simulink model "Design_of_an_Energy_Efficient_Hybrid_Electric_Vehicle"  (R2023a)
settings: Solver=FixedStepDiscrete  StartTime=0  StopTime=110  RelTol=1e-3  EnableMultiTasking=on
PreLoadFcn:
  | power_motordrive_IPMSM_FOC_data
InitFcn:
  | power_motordrive_IPMSM_FOC_data
  | Cdc  = 0.001;      % DC-link capacitor  [F]
  | AH0  = 280;        % Initial battery charge [hr*A]
  | Tmax=410;
  | 
  | %% Vehicle Parameters for Vehicle Dynamics 2
  | vehicle_mass = 2111;
  | wheel_radius = 0.228;
  | area =2.22;
  | drag_coefficient = 0.23;
  | air_density = 1.204;
  | gravity = 9.81;
  | rolling_res_ratio = 0.02;
  | 
  | % Differential drive parameters
  | gear_ratio = 5;
  | i_t   = gear_ratio ;
  | Rw=wheel_radius;
  | 
  | 
  | %% Sliding Mode Observer
  | pmsm.N_max=wmax;
  | pmsm.p=p
  | pmsm.Ld=Ld;
  | pmsm.Lq=Lq;
  | pmsm.Rs=Rs;
  | PU_System.V_base=(Vdc_nom/sqrt(3));
  | PU_System.I_base=lambda/(Lq-Ld);
  | max_torque=400
  | force_max_pedal=500
  | braking_torque_to_pedal_force_ratio=-4
undefined symbols (not defined in the file): BlkSampleTime, CurrentObserverGain, dataType, DiscIntNeverNeededParam, Fsw, gcbh, Ki_Ireg, Ki_wreg, Kp_Ireg, Kp_wreg, L_smo_gain, lambda, Ld, Limit_Ireg, Limit_wreg, Lq, MaxApplicationSpeed, MaxStatorCurrent, MaxStatorVoltage, NumBits1, NumBits2, p, Pmsm, PolePairs, QPLL, rpm_data, Sensorless, sigbuilder_block, SlidingLimit, Slope1, Slope2, sps_rtmsupport, StatorInductance, StatorResistance, Tmax_data, Tnom, Ts, Vdc_nom, wmax
libraries: fl_lib x27, nesl_utility x24, simulink x23, mcbcontrolslib x15, fl_ps_legacy_lib x9, spsStairGeneratorLib x7, sdl_lib x6, ee_lib x4, mcbpositiondecoderlib x4, BoomBox x3, tiiqmathlib x2, autolibshared x2
(part 1 of 4)
settings Model: SimulationMode=accelerator  Creator=The MathWorks, Inc.  LastModifiedBy=Dell
settings SolverCC: AlgebraicLoopSolver=TrustRegion  AutoInsertRateTranBlk=on
settings DataIOCC: SaveOutput=off  SignalLogging=off  DSMLogging=off  SaveTime=off  ReturnWorkspaceOutputs=off
settings DebuggingCC: UnconnectedInputMsg=warning  UnconnectedOutputMsg=warning  UnconnectedLineMsg=warning
settings ModelReferenceCC: EnableRefExpFcnMdlSchedulingChecks=on
settings RTWCC: DLArmComputeVersion=19.05

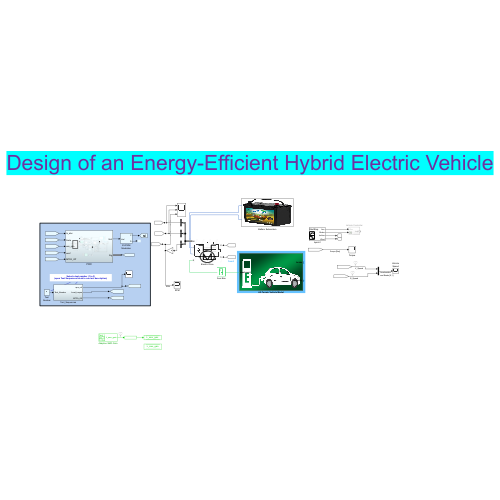
[thumbnail: Simulink's stored preview of the top-level diagram]
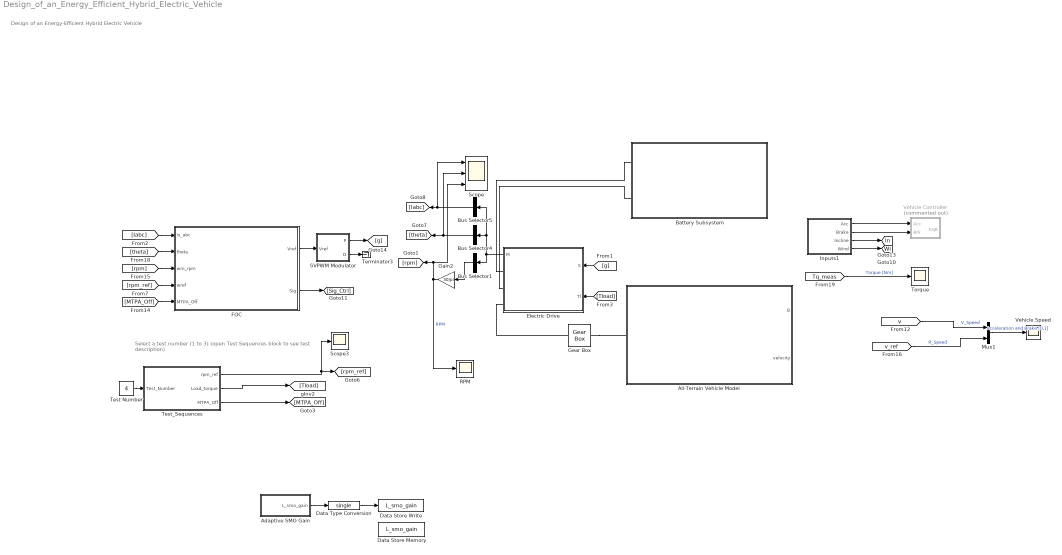
== system Design_of_an_Energy_Efficient_Hybrid_Electric_Vehicle ==
  note: Design of an Energy-Efficient Hybrid Electric Vehicle
  note: Select a test number (1 to 3)
      | (open Test Sequences block to see test description)
  Adaptive SMO Gain : Subsystem  Tag=STV Subsys  LoadFcn=sigbuilder_block('load');  StartFcn=sigbuilder_block('start');  StopFcn=sigbuilder_block('stop');  ClipboardFcn=sigbuilder_block('clipboard');  mask(Sigbuilder block){tuvar=[0:10]}
      mask help: Simulink:masks:SigbuilderBlock_MD
      mask init:
      | if ~strcmp(get_param(bdroot(gcbh),'SimulationStatus'),'stopped') tuvar = sigbuilder_block('maskInit'); end
      settings: CopyFcn=sigbuilder_block('copy');  DeleteFcn=sigbuilder_block('delete');  ModelCloseFcn=sigbuilder_block('modelClose');  PreSaveFcn=sigbuilder_block('preSave');  PauseFcn=sigbuilder_block('pause');  ContinueFcn=sigbuilder_block('continue');  NameChangeFcn=sigbuilder_block('namechange');  OpenFcn=sigbuilder_block('open',[856.5 311.25 577.5 270 ]);  CloseFcn=sigbuilder_block('close');
      mask Display: plot(0, 0, 100, 100,[2, 2, 32, 32, 2], [68, 8, 8, 68, 68],[32, 2], [38, 38], [32, 19, 2],[53, 60, 44], [32, 17, 17, 2],[16, 16, 31, 31]);txt = getActiveGroup(gcbh);text(2, 100, txt,'verticalAlignment', 'top');
  All-Terrain Vehicle Model : Subsystem
      settings: PortSchema="{\"entries\":[{\"content\":{\"sides\":[{\"content\":{\"connectorIds\":[\"LConn1\"]},\"type\":\"ConnectorPlacement.EquallySpacedRectSide\",\"uuid\":\"225ad6a8-8fc7-4595-b9ef-8c4b87b40cfe\"},{\"content\":{\"connectorIds\":[\"In1\",\"Out1\"],\"side\":\"RIGHT\"},\"type\":\"ConnectorPlacement.EquallySpacedRectSide\",\"uuid\":\"13f94d11-18ff-4ce4-b375-9246f1fbade2\"},{\"content\":{\"connectorIds\":[],\"side\":\"TOP\"},\"type\":\"ConnectorPlacement.EquallySpacedRectSide\",\"uuid\":\"c83a2beb-26a5-4534-bf12-a450c45d6815\"}]},\"type\":\"ConnectorPlacement.EquallySpacedConnector\",\"uuid\":\"18d6726c-e07c-4184-b8b4-fe9d1a75a997\"}],\"packageUris\":[\"http://schema.mathworks.com/mf0/Connector/R2020b\"],\"version\":\"1.0\"}"
      mask Display:
      | image('electric-car.png');
      | port_label('input', 1, 'brake')
      | port_label('lconn', 1 , 'mech port')
      | port_label('output', 1, 'velocity')
  Battery Subsystem : Subsystem
      mask Display: image('Battery.png'); % Use "Edit Image" on toolstrip to change.
  Bus Selector1 : BusSelector  OutputSignals=w  OutputAsBus=on
  Bus Selector4 : BusSelector  OutputSignals=A  OutputAsBus=on
  Bus Selector5 : BusSelector  OutputSignals=iabc  OutputAsBus=on
  Data Store Memory : DataStoreMemory  DataStoreName=L_smo_gain  ReadBeforeWriteMsg=warning  WriteAfterWriteMsg=warning  WriteAfterReadMsg=warning  InitialValue=0.04  ShowAdditionalParam=off
  Data Store Write : DataStoreWrite  DataStoreName=L_smo_gain  IndexOptions=Index vector (dialog)  Indices=1  OutputSizes=1
  Data Type Conversion : DataTypeConversion  OutDataTypeStr=single  SaturateOnIntegerOverflow=off  RndMeth=Floor
  Electric Drive : Subsystem  Tag=PublishSubsystem
      mask Display:
      | image('Motor.png');
      | % Circle
      | plot(sin(0:0.1:2.2*pi)*0.9,cos(0:0.1:2.2*pi)*0.9);
      | 
      | % In/out
      | plot([-1.1 -0.9],[0 0]);
      | plot([1.1 0.9],[0 0]);
      | 
      | % 'M'
      | plot([0.5 0.5],[-0.5 0.5]);
      | plot([-0.5 -0.5],[-0.5 0.5]);
      | plot([0.5 0],[0.5 -0.5]);
      | plot([-0.5 0],[0.5 -0.5]);
      | 
      | % Inputs and Outputs
      | plot([0.5 0.5],[0.9 1.8]);
      | plot([0.5 1.1],[1.8 1.8]);
      | 
      | plot([-0.5 -0.5],[0.9 1.8]);
      | plot([-0.5 -1.1],[1.8 1.8]);
      | 
      | 
      | % Plot points to set plot range
      | color('white');plot(1.9,2.8);plot(-1.9,0)
      | color('black');
  FOC : Subsystem
  Gain2 : Gain  Gain=30/pi
  Gear Box : fl_lib/Mechanical/Mechanisms/Gear Box  ratio=i_t  t_in_specify=off  t_in_priority=None  t_in=0 N*m  t_in_nominal_specify=off  t_in_nominal_unit=N*m  t_in_nominal_value=1  t_out_specify=off  t_out_priority=None  t_out=0 N*m  t_out_nominal_specify=off  t_out_nominal_unit=N*m  t_out_nominal_value=1
  Inputs1 : Subsystem  Tag=STV Subsys  LoadFcn=sigbuilder_block('load');  StartFcn=sigbuilder_block('start');  StopFcn=sigbuilder_block('stop');  ClipboardFcn=sigbuilder_block('clipboard');  mask(Sigbuilder block){tuvar=[0:10]}
      mask help: Simulink:masks:SigbuilderBlock_MD
      mask init:
      | if ~strcmp(get_param(bdroot(gcbh),'SimulationStatus'),'stopped') tuvar = sigbuilder_block('maskInit'); end
      settings: CopyFcn=sigbuilder_block('copy');  DeleteFcn=sigbuilder_block('delete');  ModelCloseFcn=sigbuilder_block('modelClose');  PreSaveFcn=sigbuilder_block('preSave');  PauseFcn=sigbuilder_block('pause');  ContinueFcn=sigbuilder_block('continue');  NameChangeFcn=sigbuilder_block('namechange');  OpenFcn=sigbuilder_block('open',[34.8 282.6 622.2 352.8 ]);  CloseFcn=sigbuilder_block('close');
      mask Display: plot(0, 0, 100, 100,[2, 2, 32, 32, 2], [68, 8, 8, 68, 68],[32, 2], [38, 38], [32, 19, 2],[53, 60, 44], [32, 17, 17, 2],[16, 16, 31, 31]);txt = getActiveGroup(gcbh);text(2, 100, txt,'verticalAlignment', 'top');
  Mux1 : Mux  Inputs=2
  RPM : Scope
  SVPWM Modulator : Subsystem  DialogController=POWERSYS.PowerSysDialog  LoadFcn=sps_rtmsupport('LoadFcn', gcbh);  StartFcn=sps_rtmsupport('StartFcn', gcbh);  StopFcn=sps_rtmsupport('StopFcn', gcbh);  mask(Unified PWM Modulator for a 2-level, 3-phase converter){PWMmethod=Space Vector PWM (SVPWM) with pulse averaging, Fsw=Fsw, Ts=Ts}
      mask prompts: PWMmethod "PWM method"; Fsw "Switching frequency (Hz):"; Ts "Sample time (s):"
      mask help:
      | Generate pulses for PWM-controlled two-level, three-phase power electronics converter with pulse averaging capability.
      |
      | The pulses generation can be perform using one of the following Pulse-Width Modulation (PWM) methods:
      | 1. Sinusoidal PWM (SPWM)
      | 2. Sinusoidal PWM (SPWM) with pulse averaging
      | 3. Space Vector PWM (SVPWM)
      | 4. Space Vector PWM (SVPWM) with pulse averaging
      | 5. 30 degrees discontinuous PWM
      |
      | When a PWM method with pulse averaging is selected, the output pulses are averaged over one sample time. (Pulses value will range from 0 to 1)
      mask init:
      | switch PWMmethod
      |     case 1 % SPWM
      |         ZeroOrderHold_Ts=-1;
      |         Pavg=0;
      |     case 2 % SPWM with pulse averaging
      |         ZeroOrderHold_Ts=-1;
      |         Pavg=1;
      |     case 3  % SVPWM
      |         ZeroOrderHold_Ts=-1;
      |         Pavg=0;
      |     case 4  % SVPWM with pulse averaging
      |         ZeroOrderHold_Ts=-1;
      |         Pavg=1;
      |     case 5  % 30 degrees discontinuous PWM
      |         ZeroOrderHold_Ts=1/Fsw/2;
      |         Pavg=0;
      | end
      settings: CopyFcn=sps_rtmsupport('CopyFcn', gcbh);  DeleteFcn=sps_rtmsupport('DeleteFcn', gcbh);  UndoDeleteFcn=sps_rtmsupport('UndoDeleteFcn', gcbh);  ModelCloseFcn=sps_rtmsupport('ModelCloseFcn', gcbh);  PreSaveFcn=sps_rtmsupport('PreSaveFcn', gcbh);  PostSaveFcn=sps_rtmsupport('PostSaveFcn', gcbh);  NameChangeFcn=sps_rtmsupport('NameChangeFcn', gcbh);  PreCopyFcn=sps_rtmsupport('PreCopyFcn', gcbh);  OpenFcn=sps_rtmsupport('OpenFcn', gcbh, [1]);  CloseFcn=sps_rtmsupport('CloseFcn', gcbh);  PreDeleteFcn=sps_rtmsupport('PreDeleteFcn', gcbh);
      mask TypeOptions PWMmethod: Sinusoidal PWM (SPWM) | Sinusoidal PWM (SPWM) wirh pulse averaging | Space Vector PWM (SVPWM) | Space Vector PWM (SVPWM) with pulse averaging | 30 degrees discontinuous PWM
  Scope : Scope  NumInputPorts=3
  Scope3 : Scope
  Terminator3 : Terminator
  Test Number : Constant  Value=4
  Test_Sequences : Subsystem
  Torque : Scope
  Vehicle Speed : Scope
  Vehicle Controller : Subsystem  Commented=on
  tag scope: In=global, Wi=global
  wires:
  [Iabc] -> FOC/1(Is_abc)
  Test Number/1 -> Test_Sequences/1(Test_Number)
  Test_Sequences/2(Load_torque) -> [Tload]
  [MTPA_Off] -> FOC/5(MTPA_Off)
  SVPWM Modulator/1(P) -> [g]
  [theta] -> FOC/2(theta)
  FOC/2(Sig) -> [Sig_Ctrl]
  Test_Sequences/1(rpm_ref) -> Scope3/1, [rpm_ref]
  [rpm] -> FOC/3(wm_rpm)
  SVPWM Modulator/2(D) -> Terminator3/1
  FOC/1(Vref) -> SVPWM Modulator/1(Vref)
  [rpm_ref] -> FOC/4(wref)
  Test_Sequences/3(MTPA_Off) -> [MTPA_Off]
  [g] -> Electric Drive/1(S)
  Electric Drive/1(M) -> Bus Selector1/1, Bus Selector5/1, Bus Selector4/1
  Bus Selector1/1 -> Gain2/1
  Bus Selector4/1 -> Scope/2, [theta]
  Bus Selector5/1 -> Scope/1, [Iabc]
  Inputs1/1(Acc) -> Vehicle Controller/1(Acc)
  Inputs1/2(Brake) -> Vehicle Controller/2(Brk)
  Inputs1/3(Incline) -> [In]
  Inputs1/4(Wind) -> [Wi]
  [v] -> Mux1/1  "V_Speed"
  [v_ref] -> Mux1/2  "R_Speed"
  Mux1/1 -> Vehicle Speed/1  "Acceleration and Brake [0,1]"
  [Tq_meas] -> Torque/1  "Torque [Nm]"
  [Tload] -> Electric Drive/2(Tl)
  Adaptive SMO Gain/1(L_smo_gain) -> Data Type Conversion/1
  Data Type Conversion/1 -> Data Store Write/1
  Gain2/1 -> Scope/3, [rpm], RPM/1  "RPM"
  connections:
  Gear Box/LConn1 -- Electric Drive/RConn3
  Gear Box/RConn1 -- All-Terrain Vehicle Model/LConn1
  Battery Subsystem/LConn1 -- Electric Drive/RConn1
  Battery Subsystem/LConn2 -- Electric Drive/RConn2

== system Design_of_an_Energy_Efficient_Hybrid_Electric_Vehicle/Adaptive SMO Gain ==
  Demux : Demux  Tag=STV Demux  Outputs=1
      settings: DisplayOption=none
  FromWs : FromWorkspace  Tag=STV FromWs  VariableName=tuvar  SampleTime=Ts
      SigBuilderData=|
      | common.afterFinalStr = 'Extrapolate'
      | common.sampleTime = 'Ts'
      | dataSet.timeRange = [0 13]
      | dataSet.name = 'Test 1'
      | sbobj.Groups.Name = 'Test 1'
      | sbobj.Groups.Signals.Name = 'L_smo_gain'
      | sbobj.Groups.Signals.XData = [0 0.7 1.3 2 3 3.5 4 4.5 5.7 6 7.5 10 13]
      | sbobj.Groups.Signals.YData = [0.02 0.02 0.02 0.02 0.17 0.17 0.17 0.17 0.17 0.17 0.095 0.095 0.1]
      | sbobj.Groups.TimeRange = [0 13]
  L_smo_gain : Outport  Tag=STV Outport  VectorParamsAs1DForOutWhenUnconnected=off
  wires:
  FromWs/1 -> Demux/1
  Demux/1 -> L_smo_gain/1

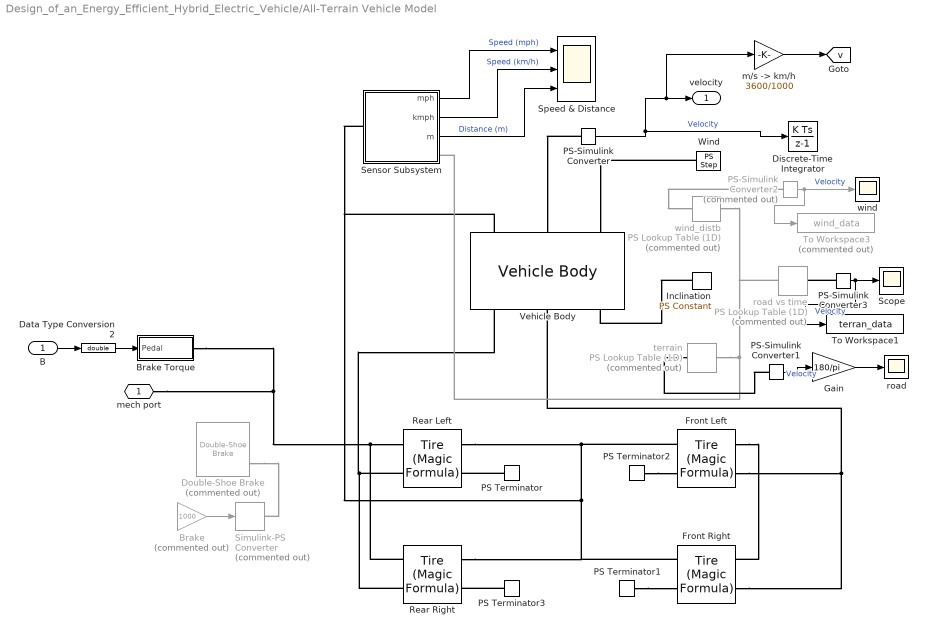
== system Design_of_an_Energy_Efficient_Hybrid_Electric_Vehicle/All-Terrain Vehicle Model ==
  B : Inport
  " Front Left" : sdl_lib/Tires & Vehicles/Tire (Magic Formula)  parameterization=2  F_z1=3000 N  F_x1=3500 N  kappa1=10  B_m=10  C_m=1.9  D_m=1  E_m=0.97  fz0=4000 N  p_Cx=1.685  p_Dx=[1.21, -.037]  p_Ex=[.344, .095, -.02, 0]  p_Kx=[21.51, -.163, .245]  p_Hx=[-.002, .002]  p_Vx=[0, 0]  rolling_radius_model=sdl.enum.RollingRadiusParameterization.Constant  r_e=wheel_radius m  r_0=0.3 m  breff=8.39  dreff=0.26  freff=0.074  q_re0=0.99  q_v1=0.008  longvl=17 m/s  cz=5e5 N/m  model_resistance=simscape.enum.onoff.on  resistance_model=1  coeff=rolling_res_ratio  p_tire=250e3 Pa  alpha=-0.003  beta=0.97  coeff_a=84e-4  coeff_b=6.2e-4 s/m  coeff_c=1.6e-4 s^2/m^2  p_tire0=240e3 Pa  fz0_resistance=4000 N  vH0=16 m/s  q_Sy=[.0082, 0, .0014, .001, 0, 0, 1.08, -.5]  v_thr=0.001 m/s  enable_scaling_coefficients=false  lfzO=1  lcx=1  lmux=1  lex=1  lkx=1  lhx=1  lvx=1  lmy=1  model_compliance=0  stiffness=1e6 N/m  damping=1000 N/(m/s)  model_inertia=1  inertia=1e-2 kg*m^2  initial_velocity=0 rpm  vxlow=0.1 m/s  v_tr_thr=0.1*(0.1) m/s  kpumin=-1e5  kpumax=1e5
  " Front Right" : sdl_lib/Tires & Vehicles/Tire (Magic Formula)  parameterization=2  F_z1=3000 N  F_x1=3500 N  kappa1=10  B_m=10  C_m=1.9  D_m=1  E_m=0.97  fz0=4000 N  p_Cx=1.685  p_Dx=[1.21, -.037]  p_Ex=[.344, .095, -.02, 0]  p_Kx=[21.51, -.163, .245]  p_Hx=[-.002, .002]  p_Vx=[0, 0]  rolling_radius_model=sdl.enum.RollingRadiusParameterization.Constant  r_e=wheel_radius m  r_0=0.3 m  breff=8.39  dreff=0.26  freff=0.074  q_re0=0.99  q_v1=0.008  longvl=17 m/s  cz=5e5 N/m  model_resistance=simscape.enum.onoff.on  resistance_model=1  coeff=rolling_res_ratio  p_tire=250e3 Pa  alpha=-0.003  beta=0.97  coeff_a=84e-4  coeff_b=6.2e-4 s/m  coeff_c=1.6e-4 s^2/m^2  p_tire0=240e3 Pa  fz0_resistance=4000 N  vH0=16 m/s  q_Sy=[.0082, 0, .0014, .001, 0, 0, 1.08, -.5]  v_thr=0.001 m/s  enable_scaling_coefficients=false  lfzO=1  lcx=1  lmux=1  lex=1  lkx=1  lhx=1  lvx=1  lmy=1  model_compliance=0  stiffness=1e6 N/m  damping=1000 N/(m/s)  model_inertia=1  inertia=1e-2 kg*m^2  initial_velocity=0 rpm  vxlow=0.1 m/s  v_tr_thr=0.1*(0.1) m/s  kpumin=-1e5  kpumax=1e5
  " Rear Left" : sdl_lib/Tires & Vehicles/Tire (Magic Formula)  parameterization=2  F_z1=3000 N  F_x1=3500 N  kappa1=10  B_m=10  C_m=1.9  D_m=1  E_m=0.97  fz0=4000 N  p_Cx=1.685  p_Dx=[1.21, -.037]  p_Ex=[.344, .095, -.02, 0]  p_Kx=[21.51, -.163, .245]  p_Hx=[-.002, .002]  p_Vx=[0, 0]  rolling_radius_model=sdl.enum.RollingRadiusParameterization.Constant  r_e=wheel_radius m  r_0=0.3 m  breff=8.39  dreff=0.26  freff=0.074  q_re0=0.99  q_v1=0.008  longvl=17 m/s  cz=5e5 N/m  model_resistance=1  resistance_model=1  coeff=rolling_res_ratio  p_tire=250e3 Pa  alpha=-0.003  beta=0.97  coeff_a=84e-4  coeff_b=6.2e-4 s/m  coeff_c=1.6e-4 s^2/m^2  p_tire0=240e3 Pa  fz0_resistance=4000 N  vH0=16 m/s  q_Sy=[.0082, 0, .0014, .001, 0, 0, 1.08, -.5]  v_thr=0.001 m/s  enable_scaling_coefficients=false  lfzO=1  lcx=1  lmux=1  lex=1  lkx=1  lhx=1  lvx=1  lmy=1  model_compliance=0  stiffness=1e6 N/m  damping=1000 N/(m/s)  model_inertia=1  inertia=1e-2 kg*m^2  initial_velocity=0 rpm  vxlow=0.1 m/s  v_tr_thr=0.1*(0.1) m/s  kpumin=-1e5  kpumax=1e5
  " Rear Right" : sdl_lib/Tires & Vehicles/Tire (Magic Formula)  parameterization=2  F_z1=3000 N  F_x1=3500 N  kappa1=10  B_m=10  C_m=1.9  D_m=1  E_m=0.97  fz0=4000 N  p_Cx=1.685  p_Dx=[1.21, -.037]  p_Ex=[.344, .095, -.02, 0]  p_Kx=[21.51, -.163, .245]  p_Hx=[-.002, .002]  p_Vx=[0, 0]  rolling_radius_model=sdl.enum.RollingRadiusParameterization.Constant  r_e=wheel_radius m  r_0=0.3 m  breff=8.39  dreff=0.26  freff=0.074  q_re0=0.99  q_v1=0.008  longvl=17 m/s  cz=5e5 N/m  model_resistance=1  resistance_model=1  coeff=rolling_res_ratio  p_tire=250e3 Pa  alpha=-0.003  beta=0.97  coeff_a=84e-4  coeff_b=6.2e-4 s/m  coeff_c=1.6e-4 s^2/m^2  p_tire0=240e3 Pa  fz0_resistance=4000 N  vH0=16 m/s  q_Sy=[.0082, 0, .0014, .001, 0, 0, 1.08, -.5]  v_thr=0.001 m/s  enable_scaling_coefficients=false  lfzO=1  lcx=1  lmux=1  lex=1  lkx=1  lhx=1  lvx=1  lmy=1  model_compliance=0  stiffness=1e6 N/m  damping=1000 N/(m/s)  model_inertia=1  inertia=1e-2 kg*m^2  initial_velocity=0 rpm  vxlow=0.1 m/s  v_tr_thr=0.1*(0.1) m/s  kpumin=-1e5  kpumax=1e5
  Brake : Gain  Commented=on  Gain=1000
  Brake Torque : Subsystem
  Data Type Conversion2 : DataTypeConversion  OutDataTypeStr=double  SaturateOnIntegerOverflow=off  RndMeth=Floor
  Discrete-Time Integrator : DiscreteIntegrator  SampleTime=-1  ICPrevOutput=DiscIntNeverNeededParam  ICPrevScaledInput=DiscIntNeverNeededParam
  Double-Shoe Brake : sdl_lib/Brakes & Detents/Rotational/Double-Shoe Brake  Commented=on  r_drum=150 mm  r_act=100 mm  r_pin=125 mm  theta_pin=15 deg  theta_0=5 deg  theta_shoe=120 deg  mu_visc=.01 N*m/(rad/s)  thermal_port=simscape.enum.thermaleffects.omit  mu=0.3  temperature_TLU=[280.0, 300.0, 320.0] K  mu_TLU=[0.1, 0.05, 0.03]  w_thr=0.01 rad/s  enable_faults=simscape.enum.onoff.off  faulted_force=0 N  external_fault=simscape.enum.onoff.off  temporal_fault=simscape.enum.onoff.off  fault_time=5 s  report_fault=simscape.enum.assert.action.none  thermal_mass=50 kJ/K  temperature_specify=off  temperature_priority=High  temperature=300 K  temperature_nominal_specify=off  temperature_nominal_unit=K  temperature_nominal_value=1
      settings: InternalSimscapePortConfiguration="{\"Bottom\":[],\"Left\":[{\"id\":\"F\",\"label\":\"F\",\"type\":\"input\"},{\"id\":\"S\",\"label\":\"S\",\"type\":\"foundation.mechanical.rotational.rotational\"}],\"Right\":[],\"Top\":[]}"
  Gain : Gain  Gain=180/pi
  Inclination : fl_lib/Physical Signals/Sources/PS Constant  constant=0
  PS Terminator{,1..3} (4 alike) : fl_lib/Physical Signals/Sinks/PS Terminator
  PS-Simulink Converter : nesl_utility/PS-Simulink Converter  PhysicalDomain=network_engine_domain  SubClassName=ps_output  LeftPortType=input  RightPortType=output  PseudoPeriodic=off  Frequencies=[]  VectorFormat=1-D array  Unit=m/s  AffineConversion=off
  PS-Simulink Converter1 : nesl_utility/PS-Simulink Converter  PhysicalDomain=network_engine_domain  SubClassName=ps_output  LeftPortType=input  RightPortType=output  PseudoPeriodic=off  Frequencies=[]  VectorFormat=1-D array  Unit=inherit  AffineConversion=off
  PS-Simulink Converter2 : nesl_utility/PS-Simulink Converter  Commented=on  PhysicalDomain=network_engine_domain  SubClassName=ps_output  LeftPortType=input  RightPortType=output  PseudoPeriodic=off  Frequencies=[]  VectorFormat=1-D array  Unit=inherit  AffineConversion=off
  PS-Simulink Converter3 : nesl_utility/PS-Simulink Converter  PhysicalDomain=network_engine_domain  SubClassName=ps_output  LeftPortType=input  RightPortType=output  PseudoPeriodic=off  Frequencies=[]  VectorFormat=1-D array  Unit=inherit  AffineConversion=off
  Scope : Scope
  Sensor Subsystem : Subsystem
  Simulink-PS Converter : nesl_utility/Simulink-PS Converter  Commented=on  PhysicalDomain=network_engine_domain  SubClassName=ps_input  LeftPortType=input  RightPortType=output  PseudoPeriodic=off  Frequencies=[]  NoiseDistribution=none  NoiseParameters=[]  Unit=N  AffineConversion=off  FilteringAndDerivatives=filter  SimscapeFilterOrder=2  InputFilterTimeConstant=0.001  UdotUserProvided=1
  Speed & Distance : Scope  NumInputPorts=3
  To Workspace1 : ToWorkspace  VariableName=terran_data  SaveFormat=Structure With Time  SampleTime=2.0000e-04
  To Workspace3 : ToWorkspace  Commented=on  VariableName=wind_data  SaveFormat=Structure With Time  SampleTime=2.0000e-04
  Vehicle Body : sdl_lib/Tires & Vehicles/Vehicle Body  mass="vehicle_mass  kg"  n_w=1  x_f=0.6 m  x_r=0.5 m  y_c=0.4 m  mass_var=simscape.enum.onoff.off  g=gravity m/s^2  liftoff_warning=0  area=area m^2  Cd=drag_coefficient  rho=air_density kg/m^3  model_pitch=0  inertia=4000 kg*m^2  suspension_model=1  k_f=1e4 N/m  b_f=1e4 N/(m/s)  k_r=1e4 N/m  b_r=1e4 N/(m/s)  k_f_TLU=[-2000, -1000, 0, 1000, 2000] N  x_f_TLU=[-.4, -.2, 0, .2, .4] m  b_f_TLU=[-200, -100, 0, 100, 200] N  v_f_TLU=[-4, -2, 0, 2, 4] m/s  k_r_TLU=[-2000, -1000, 0, 1000, 2000] N  x_r_TLU=[-.4, -.2, 0, .2, .4] m  b_r_TLU=[-200, -100, 0, 100, 200] N  v_r_TLU=[-4, -2, 0, 2, 4] m/s  interp_method=simscape.enum.interpolation.linear  extrap_method=simscape.enum.extrapolation.linear  model_hardstop=0  upper_bound_f=.25 m  lower_bound_f=-.25 m  stop_k_f=1e6 N/m  stop_b_f=150 N/(m/s)  upper_bound_r=.25 m  lower_bound_r=-.25 m  stop_k_r=1e6 N/m  stop_b_r=150 N/(m/s)  initial_pitch=0 rad  initial_pitch_rate=0 rad/s  v_specify=on  v_priority=High  v=0 m/s  v_nominal_specify=off  v_nominal_unit=m/s  v_nominal_value=1
  Wind : fl_lib/Physical Signals/Sources/PS Step  step_time=0 s  initial_value=10  final_value=10
  "m/s -> km/h" : Gain  Gain=3600/1000
  road : Scope
  road vs time : fl_ps_legacy_lib/Legacy Physical Signals/Lookup Tables/PS Lookup Table (1D)  Commented=on  x=disi_t  f=htd_t  interp_method=1  extrap_method=1
      settings: InternalSimscapePortConfiguration="{\"Bottom\":[],\"Left\":[{\"id\":\"I\",\"label\":\"x\",\"type\":\"input\"}],\"Right\":[{\"id\":\"O\",\"label\":\"f\",\"type\":\"output\"}],\"Top\":[]}"
  terrain : fl_ps_legacy_lib/Legacy Physical Signals/Lookup Tables/PS Lookup Table (1D)  Commented=on  x=disi_t  f=angle'  interp_method=1  extrap_method=1
      settings: InternalSimscapePortConfiguration="{\"Bottom\":[],\"Left\":[{\"id\":\"I\",\"label\":\"x\",\"type\":\"input\"}],\"Right\":[{\"id\":\"O\",\"label\":\"f\",\"type\":\"output\"}],\"Top\":[]}"
  wind : Scope
  wind_distb : fl_ps_legacy_lib/Legacy Physical Signals/Lookup Tables/PS Lookup Table (1D)  Commented=on  x=disi_w  f=htd_w  interp_method=1  extrap_method=1
      settings: InternalSimscapePortConfiguration="{\"Bottom\":[],\"Left\":[{\"id\":\"I\",\"label\":\"x\",\"type\":\"input\"}],\"Right\":[{\"id\":\"O\",\"label\":\"f\",\"type\":\"output\"}],\"Top\":[]}"
  mech port : PMIOPort  Side=Left
  velocity : Outport
  tag scope: v=global
  wires:
  PS-Simulink Converter/1 -> "m/s -> km/h"/1, velocity/1, Discrete-Time Integrator/1  "Velocity"
  Brake/1 -> Simulink-PS Converter/1
  Data Type Conversion2/1 -> Brake Torque/1(Pedal)
  B/1 -> Data Type Conversion2/1
  Sensor Subsystem/1(mph) -> Speed & Distance/1  "Speed (mph)"
  Sensor Subsystem/3(m) -> Speed & Distance/3  "Distance (m)"
  Sensor Subsystem/2(kmph) -> Speed & Distance/2  "Speed (km/h)"
  PS-Simulink Converter1/1 -> Gain/1  "Velocity"
  Gain/1 -> road/1
  PS-Simulink Converter2/1 -> To Workspace3/1, wind/1  "Velocity"
  PS-Simulink Converter3/1 -> To Workspace1/1, Scope/1  "Velocity"
  "m/s -> km/h"/1 -> [v]
  connections:
  " Front Left"/LConn2 -- " Front Right"/LConn2
  PS Terminator2/LConn1 -- " Front Left"/RConn1
  PS Terminator/LConn1 -- " Rear Left"/RConn1
  " Front Left"/LConn1 -- Vehicle Body/RConn2 -- " Front Right"/LConn1
  " Rear Left"/RConn2 -- " Front Right"/RConn2 -- " Rear Right"/RConn2 -- Sensor Subsystem/LConn1 -- Vehicle Body/LConn1 -- " Front Left"/RConn2
  PS-Simulink Converter/LConn1 -- Vehicle Body/LConn2
  " Rear Left"/LConn1 -- " Rear Right"/LConn1 -- Vehicle Body/RConn1
  mech port/RConn1 -- Brake Torque/RConn1 -- " Rear Right"/LConn2 -- " Rear Left"/LConn2
  Double-Shoe Brake/LConn1 -- Simulink-PS Converter/RConn1
  terrain/LConn1 -- wind_distb/LConn1 -- road vs time/LConn1 -- Sensor Subsystem/RConn1
  PS-Simulink Converter1/LConn1 -- terrain/RConn1
  PS-Simulink Converter2/LConn1 -- wind_distb/RConn1
  PS-Simulink Converter3/LConn1 -- road vs time/RConn1
  Inclination/RConn1 -- Vehicle Body/RConn3
  Wind/RConn1 -- Vehicle Body/LConn3
  PS Terminator1/LConn1 -- " Front Right"/RConn1
  PS Terminator3/LConn1 -- " Rear Right"/RConn1

== system Design_of_an_Energy_Efficient_Hybrid_Electric_Vehicle/Battery Subsystem ==
  Battery : batteryecm_lib/Battery  Vnom=Vdc_nom V  prm_dir=1  R1_dis=2 Ohm  R1_ch=2 Ohm  R1=0.001 Ohm  prm_AH=1  AH=300 hr*A  V1=V1 V  AH1=100 hr*A  prm_R2=1  R2=2000 Ohm  Tmeas=298.15 K  charge_measurement_port=simscape.enum.battery.enable.no  prm_dyn=1  Rp1=0.005 Ohm  tau1=30 s  Rp2=0.005 Ohm  tau2=30 s  Rp3=0.005 Ohm  tau3=30 s  Rp4=0.005 Ohm  tau4=30 s  Rp5=0.005 Ohm  tau5=30 s  prm_fade=1  N_fade=100  AH_fade=45 hr*A  R1_fade=2.02 Ohm  R1_ch_fade=2.02 Ohm  V1_fade=10.35 V  prm_age=1  prm_age_OCV=1  OCV_age=0.9  SOC_age=60  Tmeas_age=298.15 K  delta_time_age_vec=[0] d  temperature_age_vec=[273] K  OCV_scaling_age=2.2134e6  OCV_offset_age=1.632e6  temp_exp_age=0.515833569 V  t_exp_age=0.75  Vnom_T2=12 V  R1_T2=2.2 Ohm  R1_T2_dis=2.2 Ohm  R1_T2_ch=2.2 Ohm  V1_T2=11.4 V  R2_T2=2200 Ohm  Rp1_T2=0.005 Ohm  tau1_T2=30 s  Rp2_T2=0.005 Ohm  tau2_T2=30 s  Rp3_T2=0.005 Ohm  tau3_T2=30 s  Rp4_T2=0.005 Ohm  tau4_T2=30 s  Rp5_T2=0.005 Ohm  tau5_T2=30 s  Tmeas2=273.15 K  thermal_port=simscape.enum.thermaleffects.omit  thermal_mass=30000 J/K  i_specify=off  i_priority=None  i=0 A  i_nominal_specify=off  i_nominal_unit=A  i_nominal_value=1  v_specify=off  v_priority=None  v=0 V  v_nominal_specify=off  v_nominal_unit=V  v_nominal_value=1  charge_specify=on  charge_priority=High  charge=AH0 hr*A  charge_nominal_specify=off  charge_nominal_unit=A*hr  charge_nominal_value=1  num_cycles_specify=off  num_cycles_priority=High  num_cycles=0  num_cycles_nominal_specify=off  num_cycles_nominal_unit=1  num_cycles_nominal_value=1  temperature_specify=off  temperature_priority=High  temperature=298.15 K  temperature_nominal_specify=off  temperature_nominal_unit=K  temperature_nominal_value=1
  Current : Display
  Current Sensor : fl_lib/Electrical/Electrical Sensors/Current Sensor
  Electrical Reference : fl_lib/Electrical/Electrical Elements/Electrical Reference
  Gain : Gain  Gain=1/1000
  KW & W : Scope  NumInputPorts=2
  PS-Simulink Converter : nesl_utility/PS-Simulink Converter  PhysicalDomain=network_engine_domain  SubClassName=ps_output  LeftPortType=input  RightPortType=output  PseudoPeriodic=off  Frequencies=[]  VectorFormat=inherit  Unit=inherit  AffineConversion=off
  PS-Simulink Converter1 : nesl_utility/PS-Simulink Converter  PhysicalDomain=network_engine_domain  SubClassName=ps_output  LeftPortType=input  RightPortType=output  PseudoPeriodic=off  Frequencies=[]  VectorFormat=inherit  Unit=inherit  AffineConversion=off
  Power (KW) : Display
  Power (W) : Display
  Product : Product
  Solver Configuration : nesl_utility/Solver Configuration  PhysicalDomain=network_engine_domain  SubClassName=solver  LeftPortType=input  RightPortType=generic  Tones=[]  Harmonics=[]  SimulateNoise=off  Profile=off  UseLocalSampling=off  EnableSwitchedLinearOptims=on  FrequencyDomain=off  UseCCode=off  RelTol=0.001  AbsTol=1e-06  MinStep=1e-09  ToWorkspace=off  RevertToSquareIcSolve=off  NumHomotopyIterations=100  PhasorMode=off  PhasorModeNumHarmonics=1  ConsistencySolver=NEWTON_FTOL  IndexReductionMethod=DerivativeReplacement  DoDC=off  ResidualTolerance=1e-9  ConsistencyTolSource=GLOBAL  ConsistencyAbsTol=0.001  ConsistencyRelTol=0.001  ConsistencyTolFactor=0.001  UseLocalSolver=on  LocalSolverChoice=NE_BACKWARD_EULER_ADVANCER  ResolveIndetEquations=on  FunctionEvalNumThread=1  LocalSolverSampleTime=Ts  DoFixedCost=on  MaxNonlinIter=5  MaxModeIter=2  ComputeImpulses=off  ImpulseIterations=2  LinearAlgebra=auto  LinearAlgebraNumThread=0  EquationFormulation=NE_TIME_EF  DelaysMemoryBudget=1024  AutomaticFiltering=on  FilteringTimeConstant=0.001  PartitionStorageMethod=AS_NEEDED  PartitionMemoryBudget=1024  PartitionMethod=FAST
  Voltage : Display
  Voltage & Current : Scope
  Voltage Sensor : fl_lib/Electrical/Electrical Sensors/Voltage Sensor
  + : PMIOPort  Side=Left
  - : PMIOPort  Port=2  Side=Left
  wires:
  PS-Simulink Converter/1 -> Product/2, Current/1  "Current"
  Product/1 -> Gain/1, KW & W/2, Power (W)/1, Voltage & Current/1  "Watt (W)"
  Gain/1 -> KW & W/1, Power (KW)/1  "Power (KW)"
  PS-Simulink Converter1/1 -> Product/1, Voltage/1  "Voltage"
  connections:
  PS-Simulink Converter/LConn1 -- Current Sensor/RConn1
  Electrical Reference/LConn1 -- Voltage Sensor/RConn2 -- Battery/RConn1 -- -/RConn1 -- Solver Configuration/RConn1
  Current Sensor/LConn1 -- Voltage Sensor/LConn1 -- Battery/LConn1
  Voltage Sensor/RConn1 -- PS-Simulink Converter1/LConn1
  Current Sensor/RConn2 -- +/RConn1

== system Design_of_an_Energy_Efficient_Hybrid_Electric_Vehicle/Electric Drive ==
  S : Inport
  Tl : Inport  Port=2
  50 kw IPMSM : ee_lib/Electromechanical/Permanent Magnet/PMSM  port_option=ee.enum.threePhasePort.composite  winding_type=ee.enum.statorconnection.wye  machine_param=ee.enum.pmsm.parameterization.constant  nPolePairs=p  pmflux_param=ee.enum.pmflux.fluxlinkage  pm_flux_linkage=lambda Wb  torque_constant=0.18 N*m/A  back_emf_constant=0.18 V*s/rad  stator_param=ee.enum.statorparam.LdLqL0  Ld=Ld H  Lq=Lq H  idVec=[-200, 0, 200] A  iqVec=[-200, 0, 200] A  LdMatrix=0.0002 * ones(3, 3) H  LqMatrix=0.0002 * ones(3, 3) H  PmMatrix=0.1 * ones(3, 3) Wb  ktMatrix=0.18 * ones(3, 3) N*m/A  keMatrix=0.18 * ones(3, 3) V*s/rad  L0=0.00012184 H  Ls=0.0002 H  Lm=-0.00002 H  Ms=0.00002 H  Rs=Rs Ohm  zero_sequence=ee.enum.park.zerosequence.include  axes_param=ee.enum.rotorangle.qaxis  loss_param=ee.enum.ironloss.none  losses_oc=[0, 0, 0] W  losses_sc=[0, 0, 0] W  f_losses=60 Hz  Isc_losses=95 A  J=0 kg*m^2  lam=0 ft*lbf/(rad/s)  i_d_specify=off  i_d_priority=None  i_d=0 A  i_d_nominal_specify=off  i_d_nominal_unit=A  i_d_nominal_value=1  i_q_specify=off  i_q_priority=None  i_q=0 A  i_q_nominal_specify=off  i_q_nominal_unit=A  i_q_nominal_value=1  torque_specify=off  torque_priority=None  torque=0 N*m  torque_nominal_specify=off  torque_nominal_unit=N*m  torque_nominal_value=1  angular_velocity_specify=on  angular_velocity_priority=High  angular_velocity=0 rpm  angular_velocity_nominal_specify=off  angular_velocity_nominal_unit=rpm  angular_velocity_nominal_value=1  angular_position_specify=off  angular_position_priority=High  angular_position=0 deg  angular_position_nominal_specify=off  angular_position_nominal_unit=deg  angular_position_nominal_value=1  alpha=3.93e-3 1/K  alpha_flux=-0.001 1/K  Tmeas=298.15 K  stator_thermal_mass=100 J/K  rotor_thermal_mass=200 J/K  Rm_percent_rotor=90  Rd_percent_rotor=30  temperatureA_specify=off  temperatureA_priority=High  temperatureA=25 degC  temperatureA_nominal_specify=off  temperatureA_nominal_unit=degC  temperatureA_nominal_value=1  temperatureB_specify=off  temperatureB_priority=High  temperatureB=25 degC  temperatureB_nominal_specify=off  temperatureB_nominal_unit=degC  temperatureB_nominal_value=1  temperatureC_specify=off  temperatureC_priority=High  temperatureC=25 degC  temperatureC_nominal_specify=off  temperatureC_nominal_unit=degC  temperatureC_nominal_value=1  temperatureR_specify=off  temperatureR_priority=High  temperatureR=25 degC  temperatureR_nominal_specify=off  temperatureR_nominal_unit=degC  temperatureR_nominal_value=1
      settings: InternalSimscapePortConfiguration="{\"Bottom\":[],\"Left\":[{\"id\":\"N\",\"label\":\"~\",\"type\":\"foundation.electrical.three_phase\"},{\"id\":\"n\",\"label\":\"n\",\"type\":\"foundation.electrical.electrical\"}],\"Right\":[{\"id\":\"R\",\"label\":\"R\",\"type\":\"foundation.mechanical.rotational.rotational\"},{\"id\":\"C\",\"label\":\"C\",\"type\":\"foundation.mechanical.rotational.rotational\"}],\"Top\":[]}"
  Bus Creator : BusCreator  Inputs=4
  C : fl_lib/Electrical/Electrical Elements/Capacitor  c=Cdc F  r=1e-6 Ohm  g=0 1/Ohm  i_specify=off  i_priority=None  i=0 A  i_nominal_specify=off  i_nominal_unit=A  i_nominal_value=1  v_specify=off  v_priority=None  v=0 V  v_nominal_specify=off  v_nominal_unit=V  v_nominal_value=1  vc_specify=off  vc_priority=None  vc=Vnom V  vc_nominal_specify=off  vc_nominal_unit=V  vc_nominal_value=1
  Converter : ee_lib/Semiconductors & Converters/Converters/Converter (Three-Phase)  port_option=ee.enum.threePhasePort.composite  device_type=3  K=0  Vf=0.8 V  Ron=0.001 Ohm  Rds=0.001 Ohm  Goff=1e-5 1/Ohm  Vgt=1 V  Vgt_off=-1 V  Ih=1 A  Vth=0.5 V  diode_param=2  diode_Vf=0.8 V  diode_Ron=0.001 Ohm  diode_Goff=1e-5 1/Ohm  diode_C=50 nF  diode_iRM=-235 A  diode_iF=300 A  diode_idot=-50 A/us  diode_trr_param=1  diode_trr_factor=3  diode_trr=15 us  diode_Qrr=1.5e+3 s*uA  snubber_type=0  Cs=1e-7 F  Rs=0.1 Ohm
  Electrical Reference1 : fl_lib/Electrical/Electrical Elements/Electrical Reference
  Gate Driver : Subsystem
  Gmin : fl_lib/Electrical/Electrical Elements/Resistor  R=1e9 Ohm  i_specify=off  i_priority=High  i=0 A  i_nominal_specify=off  i_nominal_unit=A  i_nominal_value=1  v_specify=off  v_priority=High  v=0 V  v_nominal_specify=off  v_nominal_unit=V  v_nominal_value=1
  Inertia : fl_lib/Mechanical/Rotational Elements/Inertia  inertia=J kg*m^2  num_ports=foundation.enum.numPorts2.one  w_specify=off  w_priority=High  w=0 rad/s  w_nominal_specify=off  w_nominal_unit=rad/s  w_nominal_value=1  t_specify=off  t_priority=None  t=0 N*m  t_nominal_specify=off  t_nominal_unit=N*m  t_nominal_value=1
  MRRef Load : fl_lib/Mechanical/Rotational Elements/Mechanical Rotational Reference  Commented=on
  Meas I : Subsystem
      mask Display: %disp('iABC');
  Meas V : Subsystem
  Mechanical Rotational Reference2 : fl_lib/Mechanical/Rotational Elements/Mechanical Rotational Reference
  Sensor : Subsystem
      settings: PortSchema="{\"entries\":[{\"content\":{\"sides\":[{\"content\":{\"connectorIds\":[\"LConn1\"]},\"type\":\"ConnectorPlacement.EquallySpacedRectSide\",\"uuid\":\"f2751d26-46a7-477b-a593-dfc40190ce10\"},{\"content\":{\"connectorIds\":[\"RConn1\",\"Out1\",\"Out2\"],\"side\":\"RIGHT\"},\"type\":\"ConnectorPlacement.EquallySpacedRectSide\",\"uuid\":\"89cb8627-3d7a-45d5-b179-c3ca407dbe30\"},{\"content\":{\"connectorIds\":[],\"side\":\"TOP\"},\"type\":\"ConnectorPlacement.EquallySpacedRectSide\",\"uuid\":\"1c42d53e-4a07-49d5-951c-8beaa6872591\"}]},\"type\":\"ConnectorPlacement.EquallySpacedConnector\",\"uuid\":\"007778fa-5b21-46b6-a025-64688f82aaed\"}],\"packageUris\":[\"http://schema.mathworks.com/mf0/Connector/R2020b\"],\"version\":\"1.0\"}"
  Simulink-PS Converter : nesl_utility/Simulink-PS Converter  Commented=on  PhysicalDomain=network_engine_domain  SubClassName=ps_input  LeftPortType=input  RightPortType=output  PseudoPeriodic=off  Frequencies=[]  NoiseDistribution=none  NoiseParameters=[]  Unit=N*m  AffineConversion=off  FilteringAndDerivatives=zero  SimscapeFilterOrder=1  InputFilterTimeConstant=0.001  UdotUserProvided=1
  Torque Source : fl_lib/Mechanical/Mechanical Sources/Ideal Torque Source  Commented=on
  + : PMIOPort  Side=Right
  - : PMIOPort  Port=2  Side=Right
  R : PMIOPort  Port=3  Side=Right
  M : Outport  VectorParamsAs1DForOutWhenUnconnected=off
  tag scope: w_rad_s=global
  wires:
  S/1 -> Gate Driver/1(S)
  Bus Creator/1 -> M/1
  Meas I/1(iabc) -> Bus Creator/3  "iabc"
  Sensor/1(w) -> [w_rad_s], Bus Creator/1  "w"
  Sensor/2(A) -> Bus Creator/2  "A"
  Meas V/1(Vdc) -> Bus Creator/4  "vdc"
  Tl/1 -> Simulink-PS Converter/1
  connections:
  Electrical Reference1/LConn1 -- Gmin/LConn1
  Gate Driver/RConn1 -- Converter/LConn1
  Meas I/LConn1 -- Converter/LConn2
  R/RConn1 -- Sensor/RConn1 -- Inertia/LConn1
  C/LConn1 -- +/RConn1 -- Meas V/LConn1 -- Converter/RConn1
  C/RConn1 -- Meas V/RConn1 -- Converter/RConn2 -- -/RConn1
  Torque Source/RConn2 -- MRRef Load/LConn1
  Simulink-PS Converter/RConn1 -- Torque Source/RConn1
  50 kw IPMSM/RConn2 -- Mechanical Rotational Reference2/LConn1
  50 kw IPMSM/RConn1 -- Sensor/LConn1
  Meas I/RConn1 -- 50 kw IPMSM/LConn1
  Gmin/RConn1 -- 50 kw IPMSM/LConn2

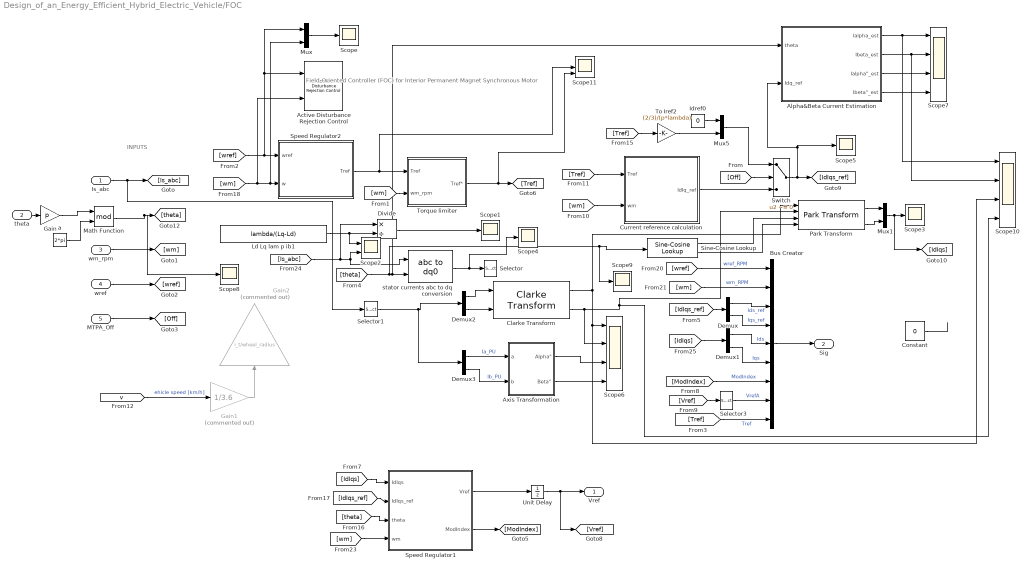
== system Design_of_an_Energy_Efficient_Hybrid_Electric_Vehicle/FOC ==
  note: INPUTS
  note: Field-Oriented Controller (FOC)
      | for
      | Interior Permanent Magnet Synchronous Motor
  Is_abc : Inport  PortDimensions=3
  theta : Inport  Port=2  PortDimensions=1
  wm_rpm : Inport  Port=3  PortDimensions=1
  wref : Inport  Port=4  PortDimensions=1
  MTPA_Off : Inport  Port=5  PortDimensions=1
  Active Disturbance Rejection Control : slctrlblks/Active Disturbance Rejection Control  time_domain=discrete-time  Ts=Ts  model_type=second-order  b0=2e7  wc=140  wo=840  x0=0  ulim_checkbox=off  umax=inf  umin=-inf  xhat_checkbox=off
  Alpha&Beta Current Estimation : Subsystem
  Axis Transformation : Subsystem  mask(Axis Transformation(120_deg)){}
  Bus Creator : BusCreator  Inputs=9
  Clarke Transform : mcbcontrolslib/Clarke Transform  VariantControl=Variant2
  Constant : Constant  Value=0
  Current reference calculation : Subsystem  mask(Current reference generation){p=p, LdLq=[Ld, Lq], lambda=lambda, Ts=Ts}
      mask prompts: p "Motor pairs of poles"; LdLq "Inductances [ Ld(H) Lq(H) ]:"; lambda "Flux linkage established by magnets (V.s)"; Ts "Sampling time (s)"
      mask init:
      | Ld=LdLq(1);
      | Lq=LdLq(2);
      | ib = lambda/(Lq-Ld);
      | Teb = 3/2*p*lambda*ib;
      | lam = lambda;
      | ib = lam/(Lq-Ld);
      | iqn = 0:0.01:3;
      | ten = iqn/2.*(sqrt(4*iqn.*iqn+1)+1);
  Demux{,1..3} (4 alike) : Demux  Outputs=2
  Divide : Product  Inputs=*/
  Gain : Gain  Gain=p
  Gain1 : Gain  Commented=on  Gain=1/3.6
  Gain2 : Gain  Commented=on  Gain=i_t/wheel_radius
  Idref0 : Constant  Value=0
  Ld Lq lam p ib1 : Constant  Value=lambda/(Lq-Ld)
  Math Function : Math  Operator=mod
  Mux : Mux  Inputs=2
  Mux1 : Mux  Inputs=2
  Mux5 : Mux  Inputs=2
  Park Transform : mcbcontrolslib/Park Transform  AxisAlignment=Q-axis
  Scope{,1,3..5,8..9} (7 alike) : Scope
  Scope10 : Scope  NumInputPorts=4
  Scope11 : Scope  NumInputPorts=3
  Scope2 : Scope  NumInputPorts=2
  Scope6 : Scope  NumInputPorts=4
  Scope7 : Scope  NumInputPorts=4
  Selector : Selector  InputPortWidth=3  IndexOptions=Index vector (dialog)  Indices=[1 2]  OutputSizes=1
  Selector1 : Selector  InputPortWidth=3  IndexOptions=Index vector (dialog)  Indices=[1 2]  OutputSizes=1
  Selector3 : Selector  InputPortWidth=3  IndexOptions=Index vector (dialog)  Indices=1  OutputSizes=1
  Sine-Cosine Lookup : mcbcontrolslib/Sine-Cosine Lookup  AngleInput=Radians  N_points=1024
  Speed Regulator1 : Subsystem  DialogController=POWERSYS.PowerSysDialog  mask(dq Current Regulators){Kp=Kp_Ireg, Ki=Ki_Ireg, Limits=Limit_Ireg, Init=0, Ts=Ts}
      mask prompts: Kp "Proportional gain (Kp):"; Ki "Integral gain (Ki):"; Limits "Output limits"; Init "Output initial value:"; Ts "Sample time:"
      mask help: This block implements dq currents regulator using anti-windup PI controllers and feedforward calculation.
      mask Display: disp('Current\nRegulators');
  Speed Regulator2 : Subsystem  DialogController=POWERSYS.PowerSysDialog  mask(Speed Regulator){Kp=Kp_wreg, Ki=Ki_wreg, Limit_wreg=Limit_wreg, Init=0, Ts=Ts}
      mask prompts: Kp "Proportional gain (Kp):"; Ki "Integral gain (Ki):"; Limit_wreg "Output limits"; Init "Output initial value:"; Ts "Sample time:"
      mask help: This block implements a speed regulator using an ant-windup PI controller.
      mask Display: disp('Speed\nRegulator');
  Switch : Switch  Criteria=u2 ~= 0  SaturateOnIntegerOverflow=off  InputSameDT=off
  To Iref2 : Gain  Gain=(2/3)/(p*lambda)
  Torque limiter : Subsystem
      mask Display: plot([0;1800;2000;2500;3000;3500], [1;1;0.90*1;0.72*1;0.6*1;0.51*1])
  Unit Delay : UnitDelay  SampleTime=-1  HasFrameUpgradeWarning=on
  a : Constant  Value=2*pi  SampleTime=-1
  stator currents abc to dq conversion : spsabctodq0Lib/abc to dq0  Alignment=90 degrees behind phase A axis
  Vref : Outport  PortDimensions=3
  Sig : Outport  Port=2
  wires:
  [wm] -> Torque limiter/2(wm_rpm)
  [Tref] -> To Iref2/1
  To Iref2/1 -> Mux5/2
  [Tref] -> Bus Creator/9  "Tref"
  Speed Regulator1/1(Vref) -> Unit Delay/1
  [Off] -> Switch/2
  MTPA_Off/1 -> [Off]
  wm_rpm/1 -> [wm]
  [ModIndex] -> Bus Creator/7  "ModIndex"
  [IdIqs_ref] -> Demux/1
  Demux/2 -> Bus Creator/4  "Iqs_ref"
  [Is_abc] -> Divide/1, Scope2/2, stator currents abc to dq conversion/1
  wref/1 -> [wref]
  stator currents abc to dq conversion/1 -> Scope4/1, Selector/1
  Switch/1 -> Alpha&Beta Current Estimation/2(Idq_ref), Scope5/1, [IdIqs_ref]
  Unit Delay/1 -> [Vref], Vref/1
  Selector3/1 -> Bus Creator/8  "VrefA"
  Idref0/1 -> Mux5/1
  Mux5/1 -> Switch/1
  theta/1 -> Gain/1
  [IdIqs] -> Speed Regulator1/1(IdIqs)
  [wm] -> Active Disturbance Rejection Control/2, Mux/2, Speed Regulator2/2(w)
  Bus Creator/1 -> Sig/1
  [theta] -> Speed Regulator1/3(theta)
  Demux/1 -> Bus Creator/3  "Ids_ref"
  [wm] -> Bus Creator/2  "wm_RPM"
  [IdIqs_ref] -> Speed Regulator1/2(IdIqs_ref)
  [IdIqs] -> Demux1/1
  [wm] -> Speed Regulator1/4(wm)
  Demux1/2 -> Bus Creator/6  "Iqs"
  [Vref] -> Selector3/1
  Demux1/1 -> Bus Creator/5  "Ids"
  Speed Regulator1/2(ModIndex) -> [ModIndex]
  Is_abc/1 -> Selector1/1, [Is_abc]
  [wref] -> Bus Creator/1  "wref_RPM"
  Math Function/1 -> Scope8/1, [theta]
  [wm] -> Current reference calculation/2(wm)
  [Tref] -> Current reference calculation/1(Tref)
  Current reference calculation/1(IdIq_ref) -> Switch/3
  Speed Regulator2/1(Tref) -> Torque limiter/1(Tref), Scope11/2
  Mux/1 -> Scope/1
  [v] -> Gain1/1  "ehicle speed [km/h]"
  Gain1/1 -> Gain2/1
  Torque limiter/1(Tref*) -> Scope11/3, [Tref]
  Ld Lq lam p ib1/1 -> Scope2/1, Divide/2
  Divide/1 -> Scope1/1
  Demux2/1 -> Clarke Transform/1
  Demux2/2 -> Clarke Transform/2
  Selector1/1 -> Demux3/1, Demux2/1
  Clarke Transform/1 -> Scope10/3, Scope6/1, Park Transform/1
  Clarke Transform/2 -> Scope6/2, Scope10/4, Park Transform/2
  Constant/1 -> ?
  Mux1/1 -> [IdIqs], Scope3/1
  Park Transform/1 -> Mux1/1
  Park Transform/2 -> Mux1/2
  Sine-Cosine Lookup/1 -> Park Transform/3
  Sine-Cosine Lookup/2 -> Park Transform/4
  Demux3/1 -> Axis Transformation/1(a)  "Ia_PU"
  Demux3/2 -> Axis Transformation/2(b)  "Ib_PU"
  Axis Transformation/2("Beta\"") -> Scope6/4
  [theta] -> Scope9/1, Sine-Cosine Lookup/1, Alpha&Beta Current Estimation/1(theta), stator currents abc to dq conversion/2
  Alpha&Beta Current Estimation/1(Ialpha_est) -> Scope10/1, Scope7/1
  Alpha&Beta Current Estimation/2(Ibeta_est) -> Scope10/2, Scope7/2
  Alpha&Beta Current Estimation/3("Ialpha\"_est") -> Scope7/3
  Alpha&Beta Current Estimation/4("Ibeta\"_est") -> Scope7/4
  Axis Transformation/1("Alpha\"") -> Scope6/3
  Gain/1 -> Math Function/1
  a/1 -> Math Function/2
  [wref] -> Mux/1, Active Disturbance Rejection Control/1, Speed Regulator2/1(wref)

== system Design_of_an_Energy_Efficient_Hybrid_Electric_Vehicle/Inputs1 ==
  Demux : Demux  Tag=STV Demux
      settings: DisplayOption=none
  FromWs : FromWorkspace  Tag=STV FromWs  VariableName=tuvar
      SigBuilderData=|
      | common.afterFinalStr = 'Extrapolate'
      | common.sampleTime = 0
      | dataSet.timeRange = [0 5]
      | dataSet.name = 'StartStop'
      | sbobj.Groups.Name = 'StartStop'
      | sbobj.Groups.Signals(1).Name = 'Acc'
      | sbobj.Groups.Signals(1).XData = [0 0.45 2 3.5 5]
      | sbobj.Groups.Signals(1).YData = [0 1 1 0 0]
      | sbobj.Groups.Signals(2).Name = 'Brake'
      | sbobj.Groups.Signals(2).XData = [0 3.6 4 5]
      | sbobj.Groups.Signals(2).YData = [0 0 0 0]
      | sbobj.Groups.Signals(3).Name = 'Incline'
      | sbobj.Groups.Signals(3).XData = [0 3.5 4 4.295 5]
      | sbobj.Groups.Signals(3).YData = [0 0 0 0 0]
      | sbobj.Groups.Signals(4).Name = 'Wind'
      | sbobj.Groups.Signals(4).XData = [0 5]
      | sbobj.Groups.Signals(4).YData = [0 0]
      | sbobj.Groups.TimeRange = [0 5]
  Acc : Outport  Tag=STV Outport  VectorParamsAs1DForOutWhenUnconnected=off
  Brake : Outport  Tag=STV Outport  Port=2  VectorParamsAs1DForOutWhenUnconnected=off
  Incline : Outport  Tag=STV Outport  Port=3  VectorParamsAs1DForOutWhenUnconnected=off
  Wind : Outport  Tag=STV Outport  Port=4  VectorParamsAs1DForOutWhenUnconnected=off
  wires:
  FromWs/1 -> Demux/1
  Demux/1 -> Acc/1
  Demux/2 -> Brake/1
  Demux/3 -> Incline/1
  Demux/4 -> Wind/1

== system Design_of_an_Energy_Efficient_Hybrid_Electric_Vehicle/SVPWM Modulator ==
  Vref : Inport  PortDimensions=3  SampleTime=Ts
  Digital Clock : DigitalClock  SampleTime=Ts
  MATLAB Function : MATLAB Function  TreatAsAtomicUnit=on
  Saturation : Saturate  UpperLimit=1  LowerLimit=0
  Zero-Order Hold : ZeroOrderHold  SampleTime=ZeroOrderHold_Ts
  P : Outport  PortDimensions=6  SampleTime=Ts  VectorParamsAs1DForOutWhenUnconnected=off
  D : Outport  Port=2  PortDimensions=3  SampleTime=Ts  VectorParamsAs1DForOutWhenUnconnected=off
  wires:
  Zero-Order Hold/1 -> MATLAB Function/1(Vref)
  Digital Clock/1 -> MATLAB Function/2(Clk)
  Saturation/1 -> P/1
  Vref/1 -> Zero-Order Hold/1
  MATLAB Function/1(P) -> Saturation/1
  MATLAB Function/2(D) -> D/1
